simulink model "differential_drive0"  (R2018a)
settings: Solver=FixedStepAuto  StartTime=0.0  StopTime=20  FixedStep=0.01  RelTol=1e-3
settings Model: EnablePacing=on  Creator=U500304  LastModifiedBy=U500304
settings SolverCC: ZeroCrossAlgorithm=Adaptive
settings DataIOCC: SaveOutput=off  SaveTime=off
settings DebuggingCC: MaxConsecutiveZCsMsg=none

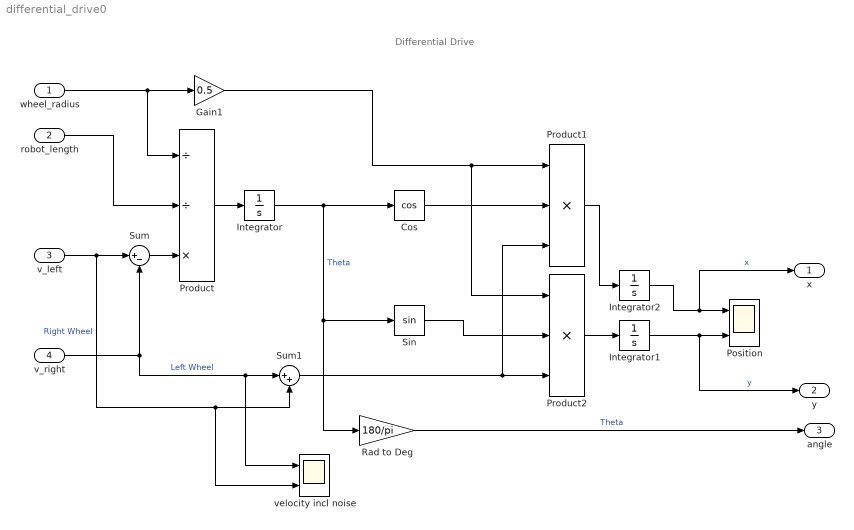
== system differential_drive0 ==
  note: Differential Drive
  wheel_radius : Inport  OutDataTypeStr=double  PortDimensions=1
  robot_length : Inport  Port=2  OutDataTypeStr=double  PortDimensions=1
  v_left : Inport  Port=3  OutDataTypeStr=double  PortDimensions=1
  v_right : Inport  Port=4  OutDataTypeStr=double  PortDimensions=1
  Cos : Trigonometry  Operator=cos
  Gain1 : Gain  Gain=0.5
  Integrator : Integrator
  Integrator1 : Integrator
  Integrator2 : Integrator
  "Position " : Scope  NumInputPorts=2
  Product : Product  Inputs=//*
  Product1 : Product  Inputs=3
  Product2 : Product  Inputs=3
  Rad to Deg : Gain  Gain=180/pi
  Sin : Trigonometry
  Sum : Sum  Inputs=|+-
  Sum1 : Sum  Inputs=|++
  velocity incl noise : Scope  NumInputPorts=2
  x : Outport  OutDataTypeStr=double  PortDimensions=1  SampleTime=0
  y : Outport  Port=2  OutDataTypeStr=double  PortDimensions=1  SampleTime=0
  angle : Outport  Port=3  OutDataTypeStr=double  PortDimensions=1  SampleTime=0
  wires:
  Gain1/1 -> Product2/1, Product1/1
  Sum/1 -> Product/3
  Integrator/1 -> Cos/1, Sin/1, Rad to Deg/1  "Theta"
  Integrator2/1 -> x/1, "Position "/1  "x"
  Cos/1 -> Product1/2
  Sum1/1 -> Product2/3, Product1/3
  v_right/1 -> Sum1/1, velocity incl noise/1, Sum/2  "Left Wheel"
  robot_length/1 -> Product/2
  Product/1 -> Integrator/1
  v_left/1 -> Sum1/2, velocity incl noise/2, Sum/1  "Right Wheel"
  Integrator1/1 -> y/1, "Position "/2  "y"
  Rad to Deg/1 -> angle/1  "Theta"
  Product2/1 -> Integrator1/1
  Product1/1 -> Integrator2/1
  wheel_radius/1 -> Gain1/1, Product/1
  Sin/1 -> Product2/2
